simulink model "triggers"  (R2023b)
settings: Solver=VariableStepAuto  StartTime=0.0  StopTime=10  RelTol=1e-3
settings Model: Creator=1234  LastModifiedBy=1234

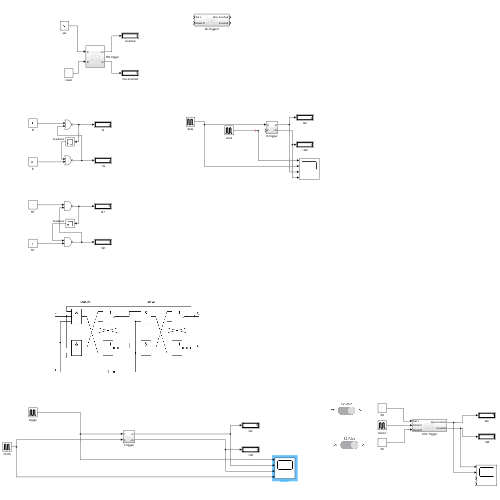
[thumbnail: Simulink's stored preview of the top-level diagram]
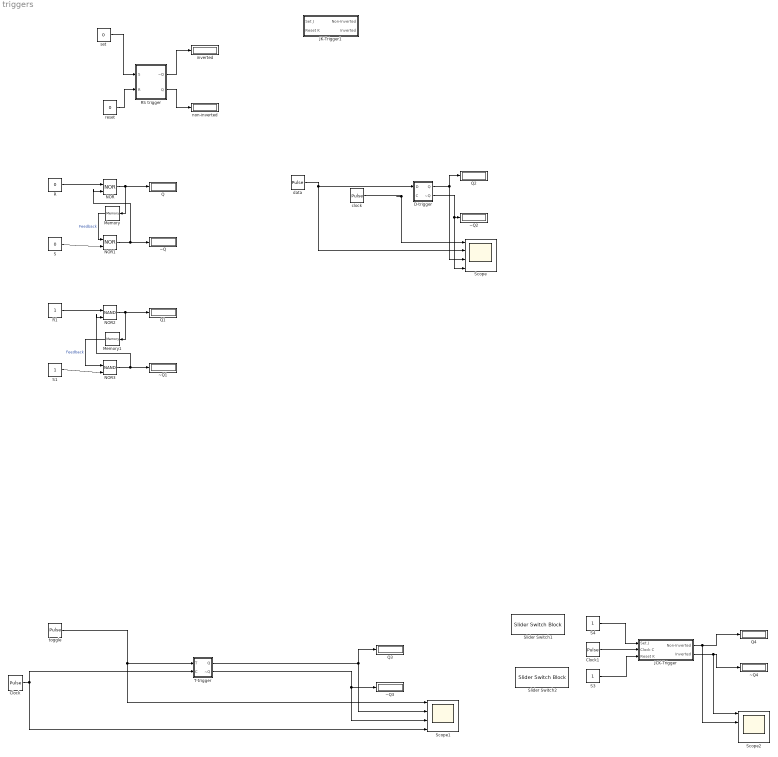
== system triggers ==
  Clock : DiscretePulseGenerator  PulseType=Time based  Period=1  PulseWidth=20
  Clock1 : DiscretePulseGenerator  PulseType=Time based  Period=1  PulseWidth=20
  D-trigger : Subsystem
  JCK-Trigger : Subsystem
  JK-Trigger1 : Subsystem
  Memory : Memory
  Memory1 : Memory
  NOR : Logic  Operator=NOR  IconShape=distinctive  AllPortsSameDT=off  OutDataTypeStr=boolean
  NOR1 : Logic  Operator=NOR  IconShape=distinctive  AllPortsSameDT=off  OutDataTypeStr=boolean
  NOR2 : Logic  Operator=NAND  IconShape=distinctive  AllPortsSameDT=off  OutDataTypeStr=boolean
  NOR3 : Logic  Operator=NAND  IconShape=distinctive  AllPortsSameDT=off  OutDataTypeStr=boolean
  Q{,1..4} (5 alike) : Display
  R : Constant  Value=0
  R1 : Constant
  RS trigger : Subsystem
  S : Constant  Value=0
  S1 : Constant
  S3 : Constant
  S4 : Constant
  Scope : Scope  NumInputPorts=4
  Scope1 : Scope  NumInputPorts=4
  Scope2 : Scope  NumInputPorts=4
  Slider Switch1 : SliderSwitchBlock
      settings: Values={{'Off', 'On'}, [0 1]}
  Slider Switch2 : SliderSwitchBlock
      settings: Values={{'Off', 'On'}, [0 1]}
  T-trigger : Subsystem
  clock : DiscretePulseGenerator  PulseType=Time based  Period=1  PulseWidth=20
  data : DiscretePulseGenerator  PulseType=Time based  Period=10  PulseWidth=20  PhaseDelay=1.5
  inverted : Display
  non-inverted : Display
  reset : Constant  Value=0
  set : Constant  Value=0
  toggle : DiscretePulseGenerator  PulseType=Time based  Period=2.5  PulseWidth=20  PhaseDelay=1
  ~Q{,1..4} (5 alike) : Display
  wires:
  set/1 -> RS trigger/1(S)
  reset/1 -> RS trigger/2(R)
  RS trigger/1(~Q) -> inverted/1
  RS trigger/2(Q) -> non-inverted/1
  S/1 -> NOR1/2
  S1/1 -> NOR3/2
  Memory1/1 -> NOR3/1  "Feedback"
  NOR3/1 -> ~Q1/1, NOR2/2
  Memory/1 -> NOR1/1  "Feedback"
  R1/1 -> NOR2/1
  NOR/1 -> Q/1, Memory/1
  NOR1/1 -> NOR/2, ~Q/1
  NOR2/1 -> Memory1/1, Q1/1
  R/1 -> NOR/1
  clock/1 -> Scope/1
  data/1 -> D-trigger/1(D), Scope/2
  D-trigger/2(~Q) -> Scope/4, ~Q2/1
  D-trigger/1(Q) -> Q2/1, Scope/3
  toggle/1 -> T-trigger/1(T), Scope1/1
  Clock/1 -> T-trigger/2(C), Scope1/4
  T-trigger/1(Q) -> Q3/1, Scope1/2
  T-trigger/2(~Q) -> Scope1/3, ~Q3/1
  Clock1/1 -> JCK-Trigger/2(Сlock C)
  S4/1 -> JCK-Trigger/1(Set J)
  S3/1 -> JCK-Trigger/3(Reset K)
  JCK-Trigger/1(Non-Inverted) -> Scope2/2, Q4/1
  JCK-Trigger/2(Inverted) -> Scope2/1, ~Q4/1

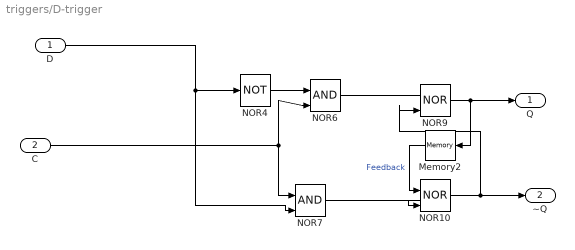
== system triggers/D-trigger ==
  D : Inport
  C : Inport  Port=2
  Memory2 : Memory
  NOR10 : Logic  Operator=NOR  IconShape=distinctive  AllPortsSameDT=off  OutDataTypeStr=boolean
  NOR4 : Logic  Operator=NOT  IconShape=distinctive  AllPortsSameDT=off  OutDataTypeStr=boolean
  NOR6 : Logic  IconShape=distinctive  AllPortsSameDT=off  OutDataTypeStr=boolean
  NOR7 : Logic  IconShape=distinctive  AllPortsSameDT=off  OutDataTypeStr=boolean
  NOR9 : Logic  Operator=NOR  IconShape=distinctive  AllPortsSameDT=off  OutDataTypeStr=boolean
  Q : Outport
  ~Q : Outport  Port=2
  wires:
  NOR10/1 -> ~Q/1, NOR9/2
  NOR9/1 -> Q/1, Memory2/1
  Memory2/1 -> NOR10/1  "Feedback"
  D/1 -> NOR7/2, NOR4/1
  NOR6/1 -> NOR9/1
  C/1 -> NOR7/1, NOR6/2
  NOR7/1 -> NOR10/2
  NOR4/1 -> NOR6/1

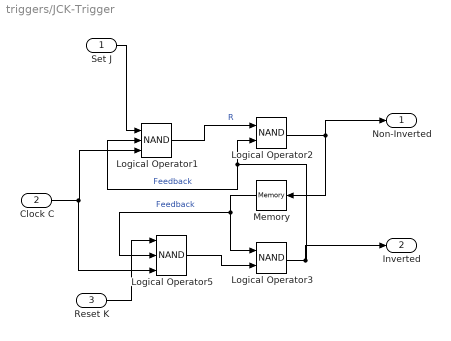
== system triggers/JCK-Trigger ==
  Set J : Inport
  Сlock C : Inport  Port=2
  Reset K : Inport  Port=3
  Logical Operator1 : Logic  Operator=NAND  Inputs=3  AllPortsSameDT=off  OutDataTypeStr=boolean
  Logical Operator2 : Logic  Operator=NAND  AllPortsSameDT=off  OutDataTypeStr=boolean
  Logical Operator3 : Logic  Operator=NAND  AllPortsSameDT=off  OutDataTypeStr=boolean
  Logical Operator5 : Logic  Operator=NAND  Inputs=3  AllPortsSameDT=off  OutDataTypeStr=boolean
  Memory : Memory
  Non-Inverted : Outport
  Inverted : Outport  Port=2
  wires:
  Memory/1 -> Logical Operator3/1, Logical Operator5/2  "Feedback"
  Logical Operator1/1 -> Logical Operator2/1  "R"
  Logical Operator2/1 -> Non-Inverted/1, Memory/1
  Logical Operator3/1 -> Inverted/1, Logical Operator1/2, Logical Operator2/2  "Feedback"
  Logical Operator5/1 -> Logical Operator3/2
  Set J/1 -> Logical Operator1/1
  Reset K/1 -> Logical Operator5/1
  Сlock C/1 -> Logical Operator5/3, Logical Operator1/3

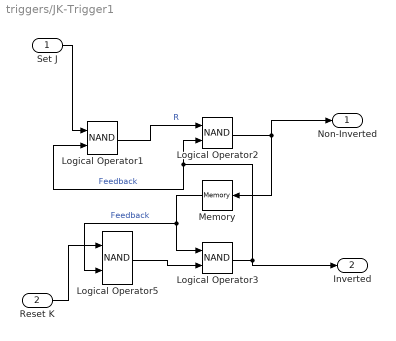
== system triggers/JK-Trigger1 ==
  Set J : Inport
  Reset K : Inport  Port=2
  Logical Operator{1..3,5} (4 alike) : Logic  Operator=NAND  AllPortsSameDT=off  OutDataTypeStr=boolean
  Memory : Memory
  Non-Inverted : Outport
  Inverted : Outport  Port=2
  wires:
  Reset K/1 -> Logical Operator5/1
  Set J/1 -> Logical Operator1/1
  Logical Operator5/1 -> Logical Operator3/2
  Logical Operator3/1 -> Logical Operator2/2, Logical Operator1/2, Inverted/1  "Feedback"
  Logical Operator2/1 -> Memory/1, Non-Inverted/1
  Logical Operator1/1 -> Logical Operator2/1  "R"
  Memory/1 -> Logical Operator3/1, Logical Operator5/2  "Feedback"

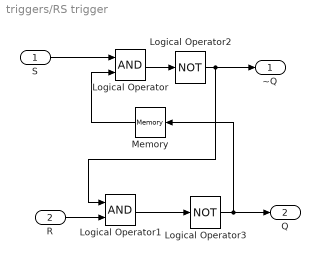
== system triggers/RS trigger ==
  S : Inport
  R : Inport  Port=2
  Logical Operator : Logic  AllPortsSameDT=off  OutDataTypeStr=boolean
  Logical Operator1 : Logic  AllPortsSameDT=off  OutDataTypeStr=boolean
  Logical Operator2 : Logic  Operator=NOT  AllPortsSameDT=off  OutDataTypeStr=boolean
  Logical Operator3 : Logic  Operator=NOT  AllPortsSameDT=off  OutDataTypeStr=boolean
  Memory : Memory
  ~Q : Outport
  Q : Outport  Port=2
  wires:
  Logical Operator3/1 -> Q/1, Memory/1
  Logical Operator2/1 -> ~Q/1, Logical Operator1/1
  S/1 -> Logical Operator/1
  Logical Operator1/1 -> Logical Operator3/1
  R/1 -> Logical Operator1/2
  Memory/1 -> Logical Operator/2
  Logical Operator/1 -> Logical Operator2/1

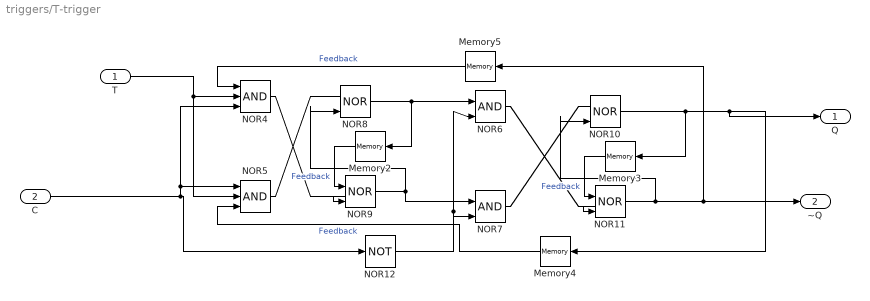
== system triggers/T-trigger ==
  T : Inport
  C : Inport  Port=2
  Memory{2..5} (4 alike) : Memory
  NOR{8..11} (4 alike) : Logic  Operator=NOR  IconShape=distinctive  AllPortsSameDT=off  OutDataTypeStr=boolean
  NOR12 : Logic  Operator=NOT  IconShape=distinctive  AllPortsSameDT=off  OutDataTypeStr=boolean
  NOR4 : Logic  Inputs=3  IconShape=distinctive  AllPortsSameDT=off  OutDataTypeStr=boolean
  NOR5 : Logic  Inputs=3  IconShape=distinctive  AllPortsSameDT=off  OutDataTypeStr=boolean
  NOR6 : Logic  IconShape=distinctive  AllPortsSameDT=off  OutDataTypeStr=boolean
  NOR7 : Logic  IconShape=distinctive  AllPortsSameDT=off  OutDataTypeStr=boolean
  Q : Outport
  ~Q : Outport  Port=2
  wires:
  Memory2/1 -> NOR9/1  "Feedback"
  NOR9/1 -> NOR8/2, NOR7/1
  NOR8/1 -> NOR6/1, Memory2/1
  NOR11/1 -> ~Q/1, Memory5/1, NOR10/2
  T/1 -> NOR5/2, NOR4/2
  NOR5/1 -> NOR8/1
  NOR12/1 -> NOR6/2, NOR7/2
  NOR10/1 -> Q/1, Memory4/1, Memory3/1
  Memory4/1 -> NOR5/3  "Feedback"
  NOR6/1 -> NOR11/2
  NOR7/1 -> NOR10/1
  Memory3/1 -> NOR11/1  "Feedback"
  C/1 -> NOR12/1, NOR4/3, NOR5/1
  NOR4/1 -> NOR9/2
  Memory5/1 -> NOR4/1  "Feedback"
